simulink model "Gemelo_Digital_RT_5_8_sincronizacion"  (R2025a)
settings: Solver=ode4  StartTime=0.0  StopTime=60  FixedStep=0.002  RelTol=1e-3  EnableMultiTasking=on
PreLoadFcn:
  | d=fileparts(get_param('Gemelo_Digital_RT_5_8_sincronizacion','FileName')); while ~isempty(d)&&~isfile(fullfile(d,'setup_paths.m')), n=fileparts(d); if strcmp(n,d),break;end; d=n; end; if isfile(fullfile(d,'setup_paths.m')), addpath(d); setup_paths; end
  | Ensamblaje_pendulo_furuta_multibody_v4_DataFile;
InitFcn:
  | Ensamblaje_pendulo_furuta_multibody_v4_DataFile;
undefined symbols (not defined in the file): Ksync_tau, tau
libraries: fl_lib x7, nesl_utility x7, sm_lib x2, ee_lib x1, quarc_library x1
settings Model: ExtModeTrigDuration=10000  Creator=sebas  LastModifiedBy=sebas
settings SolverCC: AlgebraicLoopSolver=TrustRegion  PositivePriorityOrder=on
settings DataIOCC: ReturnWorkspaceOutputs=off
settings DebuggingCC: UnconnectedInputMsg=warning  UnconnectedOutputMsg=warning  UnconnectedLineMsg=warning  ArithmeticOperatorsInVariantConditions=warning
settings ModelReferenceCC: EnableRefExpFcnMdlSchedulingChecks=on
settings SFSimCC: SimUseLocalCustomCode=off  CustomCodeUndefinedFunction=UseInterfaceOnly
settings RTWCC: SystemTargetFile=quarc_win64.tlc  TemplateMakefile=quarc_default_tmf  RTWUseLocalCustomCode=off  Toolchain=QUARC win64 | nmake (64-bit Windows)  BuildConfiguration=Faster Runs  GPUComputeCapability=3.5  Description=QUARC Win64 Target Using Toolchain
settings CodeAppCC: StateflowObjectComments=on
settings STFCustomTargetCC: SystemTargetFile=quarc_win64.tlc  TargetLangStandard=C99 (ISO)  MultiwordLength=2048.0  DynamicStringBufferSize=256.0  ConcurrentExecutionCompliant=on  UseToolchainInfoCompliant=on
settings ConfigComp: CovMetricSettings=dswe
settings ExplorerConfigSet: InternalSimMechanicsExplorerSettings="<ExplorerConfiguration><canonicalview>planar_xy</canonicalview><TilePanel><TileInfo><Tiles Columns=\"1\" Count=\"1\" Height=\"664\" Rows=\"1\" Width=\"1142\"><Row Weight=\"1\"/><Column Weight=\"1\"/><Tile Height=\"1\" Width=\"1\" X=\"0\" Y=\"0\"/></Tiles></TileInfo><SceneInfo><SceneViewer><IsThisViewStd><IsStandardView>off</IsStandardView><StandardViewName>Front</StandardViewName></IsThisViewStd><BGColor><R>1</R><G>1</G><B>1</B><A>1</A></BGColor><Camera><DoPerspective>off</DoPerspective><Position><X>0.4114893352501508</X><Y>0.5074009533335343</Y><Z>0.46019499434767086</Z></Position><Center><X>-0.027636618037190031</X><Y>0.068275000046193607</Y><Z>0.021069041060330196</Z></Center><Up><X>-0.40824829046386291</X><Y>0.81649658092772603</Y><Z>-0.40824829046386302</Z></Up><XLim>0.12087387738053319</XLim><YLim>0.12087387738053319</YLim><ViewLimDist>0.01</ViewLimDist></Camera></SceneViewer></SceneInfo></TilePanel><MechEditorPanel><GfxPanelCameraMap/><Cameras/><VideoCreator><IncludeTiles>All</IncludeTiles><IncludeTime>on</IncludeTime><IncludeWorldFrame>off</IncludeWorldFrame><PlaybackSpeedRatio>1</PlaybackSpeedRatio><FrameRate>30</FrameRate><FrameSize>auto</FrameSize><VideoFormat>UncompressedAVI</VideoFormat></VideoCreator></MechEditorPanel><PlaybackSettings><PlaybackSpeedFactor>1</PlaybackSpeedFactor></PlaybackSettings></ExplorerConfiguration>"

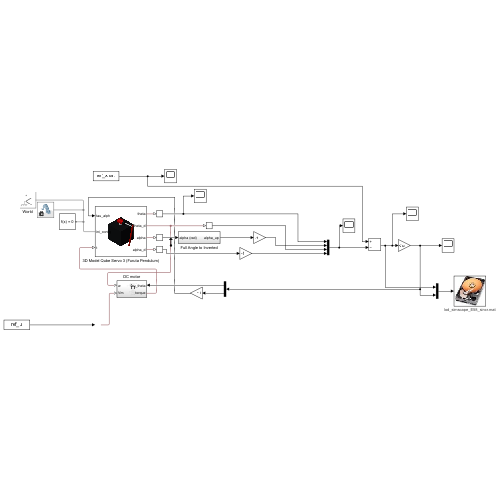
[thumbnail: Simulink's stored preview of the top-level diagram]
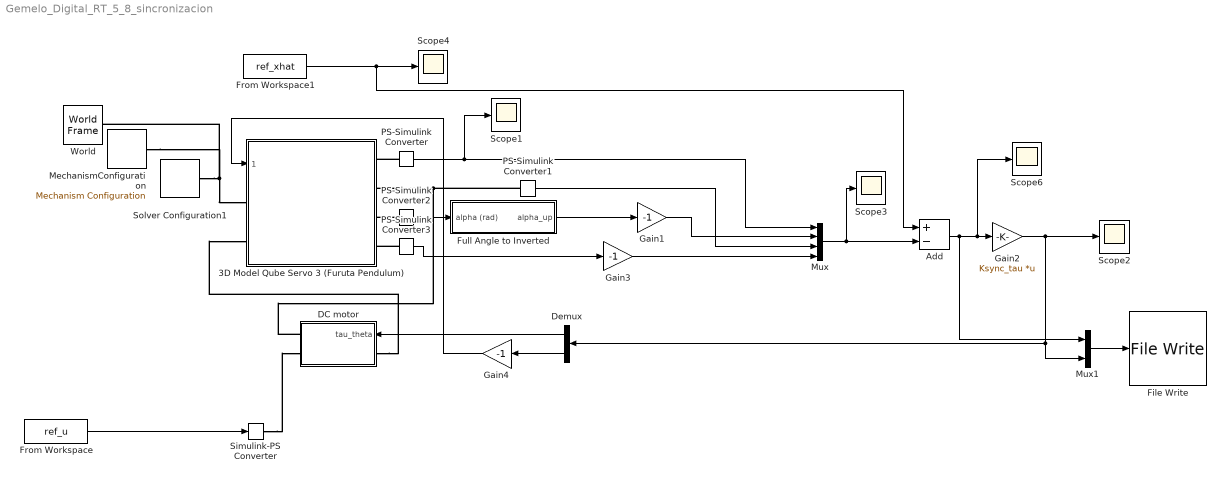
== system Gemelo_Digital_RT_5_8_sincronizacion ==
  3D Model Qube Servo 3 (Furuta Pendulum) : Subsystem  ReferencedSubsystem=Model3d_Furuta_Pendulum
  Add : Sum  Inputs=+-
  DC motor : Subsystem
  Demux : Demux  Outputs=2
  File Write : quarc_library/Sinks/To Target/File Write  source=Specify via dialog (do not evaluate)  file_name=lod_simscape_E58_sincr.mat  variable_name=error,tau  decimation=1  sample_time=-1  file_format=MAT-file v.4  options=No header or footer  append=off  encoding=Default  bitrate=0
      settings: AttributesFormatString=%<file_name>  SourceProductName=QUARC Targets
  From Workspace : FromWorkspace  VariableName=ref_u  SampleTime=0.002
  From Workspace1 : FromWorkspace  VariableName=ref_xhat  SampleTime=0.002
  Full Angle to Inverted : Subsystem
  Gain1 : Gain  Gain=-1
  Gain2 : Gain  Gain=Ksync_tau  Multiplication=Matrix(K*u)
  Gain3 : Gain  Gain=-1
  Gain4 : Gain  Gain=-1
  MechanismConfiguration : sm_lib/Utilities/Mechanism Configuration  UniformGravity=Constant  GravityVector=[0 -9.7807 0]  GravityVectorUnits=m/s^2  LinearizationDelta=0.001  JointModeTransitionNonlinearIterations=2
  Mux : Mux
  Mux1 : Mux  Inputs=2
  PS-Simulink Converter{,1..3} (4 alike) : nesl_utility/PS-Simulink Converter  PhysicalDomain=network_engine_domain  SubClassName=ps_output  LeftPortType=input  RightPortType=output  PseudoPeriodic=off  Frequencies=[]  VectorFormat=inherit  Unit=inherit  AffineConversion=off
  Scope{1..4,6} (5 alike) : Scope
      Scope1 settings: ActiveDisplayYMinimum=-2.4913575339760294  ActiveDisplayYMaximum=1.4670140162925454
      Scope2 settings: ActiveDisplayYMinimum=-1.4029766421864744  ActiveDisplayYMaximum=1.3236318563865415  DataLoggingVariableName=ScopeData2
      Scope3 settings: ActiveDisplayYMinimum=-53.363734595140478  ActiveDisplayYMaximum=47.48010473608133
      Scope4 settings: ActiveDisplayYMinimum=-37.387028597005653  ActiveDisplayYMaximum=35.963568137472  DataLoggingVariableName=ScopeData3
      Scope6 settings: ActiveDisplayYMinimum=-43.410155460919817  ActiveDisplayYMaximum=20.807441835667387  DataLoggingVariableName=ScopeData5
  Simulink-PS Converter : nesl_utility/Simulink-PS Converter  PhysicalDomain=network_engine_domain  SubClassName=ps_input  LeftPortType=input  RightPortType=output  PseudoPeriodic=off  Frequencies=[]  NoiseDistribution=none  NoiseParameters=[]  Unit=1  AffineConversion=off  FilteringAndDerivatives=filter  SimscapeFilterOrder=1  InputFilterTimeConstant=0.001  UdotUserProvided=0
  Solver Configuration1 : nesl_utility/Solver Configuration  PhysicalDomain=network_engine_domain  SubClassName=solver  LeftPortType=input  RightPortType=generic  Tones=[]  Harmonics=[]  SimulateNoise=off  Profile=off  UseLocalSampling=off  EnableSwitchedLinearOptims=on  FrequencyDomain=off  UseCCode=off  RelTol=0.001  AbsTol=0.001  MinStep=1e-09  ToWorkspace=off  RevertToSquareIcSolve=off  NumHomotopyIterations=100  PhasorMode=off  PhasorModeNumHarmonics=1  ConsistencySolver=NEWTON_XTOL_AFTER_FTOL  IndexReductionMethod=DerivativeReplacement  DoDC=off  ResidualTolerance=1e-09  ConsistencyTolSource=GLOBAL  ConsistencyAbsTol=0.001  ConsistencyRelTol=0.001  ConsistencyTolFactor=1e-9  UseLocalSolver=on  LocalSolverChoice=NE_BACKWARD_EULER_ADVANCER  ResolveIndetEquations=on  FunctionEvalNumThread=1  LocalSolverSampleTime=0.002  DoFixedCost=on  MaxNonlinIter=5  MaxModeIter=2  ComputeImpulses=on  ImpulseIterations=2  LinearAlgebra=auto  LinearAlgebraNumThread=0  EquationFormulation=NE_TIME_EF  DelaysMemoryBudget=1024  AutomaticFiltering=on  FilteringTimeConstant=0.001  PartitionStorageMethod=AS_NEEDED  PartitionMemoryBudget=1024  PartitionMethod=ROBUST  MultibodyUseLocalSolver=off  MultibodyLocalSolverChoice=ODE1  MultibodyLocalSolverSampleTime=0.002
  World : sm_lib/Frames and Transforms/World Frame
  wires:
  PS-Simulink Converter2/1 -> Full Angle to Inverted/1(alpha (rad))
  Full Angle to Inverted/1(alpha_up) -> Gain1/1
  From Workspace/1 -> Simulink-PS Converter/1
  PS-Simulink Converter3/1 -> Gain3/1
  From Workspace1/1 -> Add/1, Scope4/1
  Gain1/1 -> Mux/2
  Mux/1 -> Scope3/1, Add/2
  Gain2/1 -> Scope2/1, Demux/1, Mux1/2
  Add/1 -> Mux1/1, Scope6/1, Gain2/1
  Demux/2 -> Gain4/1
  Demux/1 -> DC motor/1(tau_theta)
  PS-Simulink Converter/1 -> Mux/1, Scope1/1
  PS-Simulink Converter1/1 -> Mux/3
  Gain3/1 -> Mux/4
  Gain4/1 -> 3D Model Qube Servo 3 (Furuta Pendulum)/1
  Mux1/1 -> File Write/1
  connections:
  Solver Configuration1/RConn1 -- MechanismConfiguration/RConn1 -- World/RConn1 -- 3D Model Qube Servo 3 (Furuta Pendulum)/LConn1
  PS-Simulink Converter2/LConn1 -- 3D Model Qube Servo 3 (Furuta Pendulum)/RConn3
  DC motor/RConn1 -- PS-Simulink Converter1/LConn1 -- 3D Model Qube Servo 3 (Furuta Pendulum)/RConn2
  PS-Simulink Converter3/LConn1 -- 3D Model Qube Servo 3 (Furuta Pendulum)/RConn4
  Simulink-PS Converter/RConn1 -- DC motor/RConn2
  PS-Simulink Converter/LConn1 -- 3D Model Qube Servo 3 (Furuta Pendulum)/RConn1
  DC motor/LConn1 -- 3D Model Qube Servo 3 (Furuta Pendulum)/LConn2

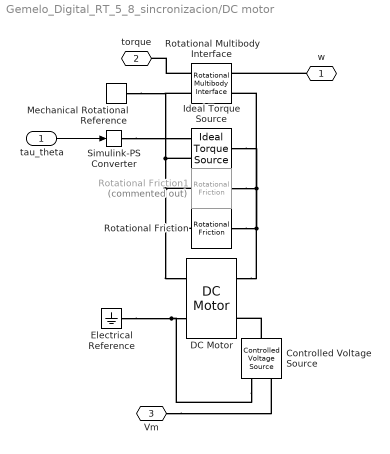
== system Gemelo_Digital_RT_5_8_sincronizacion/DC motor ==
  tau_theta : Inport
  Controlled Voltage Source : fl_lib/Electrical/Electrical Sources/Controlled Voltage Source
  DC Motor : ee_lib/Electromechanical/Brushed Motors/DC Motor  field_option=ee.enum.field_option.pm  Rf=100 Ohm  Lf=1 H  Laf=0.15 H  If0=0 A  parameterization=ee.enum.dcparam_option.circuit_param  Ra=7.5 Ohm  La=1.15e-3 H  emf_or_torque=ee.enum.emf_or_torque.kv  Kv=0.0422 V*s/rad  Ki=0.0422 N*m/A  T_stall=0.24e-3 N*m  w_max=5400 rpm  w_rated=4579 rpm  P_rated=9.8 W  V_rated=24 V  lam_param=ee.enum.lam_param.damping  i_noload=16 mA  V_i_noload=24 V  J=1.4e-6 kg*m^2  lam=1*4.8390e-6 N*m*s/rad  speed0=0 rpm  alpha=3.93e-3 1/K  Tmeas=25 degC  thermal_mass=100 J/K  initial_temperature=25 degC
  Electrical Reference : fl_lib/Electrical/Electrical Elements/Electrical Reference
  Ideal Torque Source : fl_lib/Mechanical/Mechanical Sources/Ideal Torque Source
  Mechanical Rotational Reference : fl_lib/Mechanical/Rotational Elements/Mechanical Rotational Reference
  Rotational Friction : fl_lib/Mechanical/Rotational Elements/Rotational Friction  brkwy_trq=1*2.910555e-05+1*4.081637e-05 N*m  brkwy_vel=1.082312e-02 rad/s  Col_trq=2.910555e-05 N*m  visc_coef=4.321929e-06 N*m*s/rad  w_specify=off  w_priority=None  w=0 rad/s  w_nominal_specify=off  w_nominal_value=1  w_nominal_unit=rad/s  t_specify=off  t_priority=None  t=0 N*m  t_nominal_specify=off  t_nominal_value=1  t_nominal_unit=N*m
  Rotational Friction1 : fl_lib/Mechanical/Rotational Elements/Rotational Friction  Commented=on  brkwy_trq=7.066e-04 N*m  brkwy_vel=0.1 rad/s  Col_trq=7.066e-09 N*m  visc_coef=0 N*m*s/rad  w_specify=off  w_priority=None  w=0 rad/s  w_nominal_specify=off  w_nominal_value=1  w_nominal_unit=rad/s  t_specify=off  t_priority=None  t=0 N*m  t_nominal_specify=off  t_nominal_value=1  t_nominal_unit=N*m
  Rotational Multibody Interface : fl_lib/Mechanical/Multibody Interfaces/Rotational Multibody Interface
  Simulink-PS Converter : nesl_utility/Simulink-PS Converter  PhysicalDomain=network_engine_domain  SubClassName=ps_input  LeftPortType=input  RightPortType=output  PseudoPeriodic=off  Frequencies=[]  NoiseDistribution=none  NoiseParameters=[]  Unit=1  AffineConversion=off  FilteringAndDerivatives=filter  SimscapeFilterOrder=1  InputFilterTimeConstant=0.001  UdotUserProvided=0
  w : PMIOPort  Side=Right
  torque : PMIOPort  Port=2  Side=Left
  Vm : PMIOPort  Port=3  Side=Right
  wires:
  tau_theta/1 -> Simulink-PS Converter/1
  connections:
  Rotational Friction/LConn1 -- Rotational Friction1/LConn1 -- Ideal Torque Source/LConn1 -- Rotational Multibody Interface/RConn2 -- DC Motor/LConn2
  Rotational Friction/RConn1 -- Ideal Torque Source/RConn2 -- Rotational Multibody Interface/LConn2 -- Mechanical Rotational Reference/LConn1 -- Rotational Friction1/RConn1 -- DC Motor/RConn2
  Vm/RConn1 -- Controlled Voltage Source/RConn1
  w/RConn1 -- Rotational Multibody Interface/RConn1
  DC Motor/RConn1 -- Electrical Reference/LConn1 -- Controlled Voltage Source/RConn2
  Controlled Voltage Source/LConn1 -- DC Motor/LConn1
  Rotational Multibody Interface/LConn1 -- torque/RConn1
  Simulink-PS Converter/RConn1 -- Ideal Torque Source/RConn1

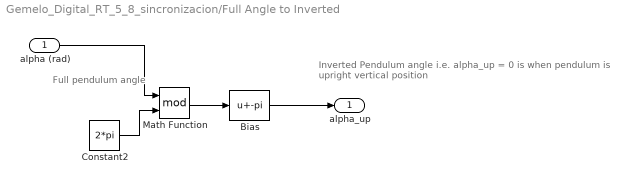
== system Gemelo_Digital_RT_5_8_sincronizacion/Full Angle to Inverted ==
  note: Full pendulum angle
  note: Inverted Pendulum angle
      | i.e. alpha_up = 0 is when pendulum is upright vertical position
  alpha (rad) : Inport
  Bias : Bias  Bias=-pi  SaturateOnIntegerOverflow=off
  Constant2 : Constant  Value=2*pi
  Math Function : Math  Operator=mod  SignedPower=on
  alpha_up : Outport  VectorParamsAs1DForOutWhenUnconnected=off
  wires:
  Math Function/1 -> Bias/1
  Bias/1 -> alpha_up/1
  Constant2/1 -> Math Function/2
  alpha (rad)/1 -> Math Function/1
